simulink model "LQR_simulation"  (R2020b)
settings: Solver=ode45  StartTime=0.0  StopTime=10  FixedStep=0.00001  RelTol=1e-3  EnableMultiTasking=on
values from neighbouring files (symbols this model uses):
  K = lqr(A, B, Q, R)    [LQR.m]
  Theta1_0 = 0    [LQR.m]    (also in LQR_discrete.m; simulation.m = 3.14159265359)
  Theta2_0 = 0.048    [LQR.m]    (also in LQR_discrete.m = 0.04; simulation.m = -1.57079632679)
  Thetad1_0 = 0    [LQR.m]    (also in LQR_discrete.m; simulation.m)
  Thetad2_0 = 0    [LQR.m]    (also in LQR_discrete.m; simulation.m)
settings Model: Creator=rbabuska  LastModifiedBy=fballast
settings DataIOCC: LimitDataPoints=on  SaveFormat=Array  ReturnWorkspaceOutputs=off  SignalLoggingName=sigsOut
settings OptimizationCC: BooleanDataType=off  ExpressionDepthLimit=2147483647  InitFltsAndDblsToZero=on  LifeSpan=inf
settings DebuggingCC: SaveWithParameterizedLinksMsg=none  SignalResolutionControl=TryResolveAllWithWarning  MultiTaskDSMMsg=warning  MultiTaskCondExecSysMsg=none  AllowSymbolicDim=off  StateNameClashWarn=warning  SFUnexpectedBacktrackingDiag=warning  SFNoUnconditionalDefaultTransitionDiag=warning  SFExecutionAtInitializationDiag=none  ArithmeticOperatorsInVariantConditions=warning
settings HardwareCC: ProdBitPerPointer=32  ProdBitPerSizeT=32  ProdBitPerPtrDiffT=32  ProdLargestAtomicFloat=None  ProdIntDivRoundTo=Undefined  ProdEndianess=Unspecified  ProdWordSize=32  ProdHWDeviceType=32-bit Generic  TargetUnknown=on
settings ModelReferenceCC: PropagateSignalLabelsOutOfModel=off
settings SFSimCC: SimUseLocalCustomCode=off  CustomCodeUndefinedFunction=UseInterfaceOnly
settings RTWCC: RTWUseLocalCustomCode=off
settings CodeAppCC: StateflowObjectComments=on
settings GRTTargetCC: TargetFcnLib=ansi_tfl_tmw.mat  TargetLangStandard=C89/C90 (ANSI)  CombineOutputUpdateFcns=off  GRTInterface=on
settings ConfigComp: CovMetricSettings=dw  CovSaveCumulativeToWorkspaceVar=on  CovSaveSingleToWorkspaceVar=on  CovExternalEMLEnable=off

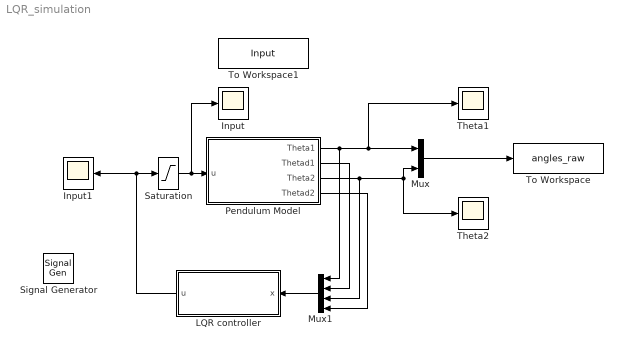
== system LQR_simulation ==
  Input : Scope
  Input1 : Scope
  LQR controller : Subsystem
  Mux : Mux  Inputs=2
  Mux1 : Mux
  Pendulum Model : Subsystem
  Saturation : Saturate  UpperLimit=1  LowerLimit=-1
  Signal Generator : SignalGenerator  Amplitude=0.7  Frequency=3  Units=rad/sec
  Theta1 : Scope
  Theta2 : Scope
  To Workspace : ToWorkspace  VariableName=angles_raw  SaveFormat=Timeseries  SampleTime=-1
  To Workspace1 : ToWorkspace  VariableName=Input  SaveFormat=Timeseries  SampleTime=-1
  wires:
  Pendulum Model/3(Theta2) -> Mux1/3, Mux/2, Theta2/1
  Mux/1 -> To Workspace/1
  Pendulum Model/1(Theta1) -> Mux1/1, Mux/1, Theta1/1
  Pendulum Model/2(Thetad1) -> Mux1/2
  Pendulum Model/4(Thetad2) -> Mux1/4
  Mux1/1 -> LQR controller/1(x)
  LQR controller/1(u) -> Saturation/1, Input1/1
  Saturation/1 -> Input/1, Pendulum Model/1(u)

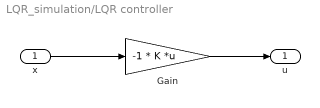
== system LQR_simulation/LQR controller ==
  x : Inport
  Gain : Gain  Gain=-1 * K  Multiplication=Matrix(K*u) (u vector)
  u : Outport
  wires:
  x/1 -> Gain/1
  Gain/1 -> u/1

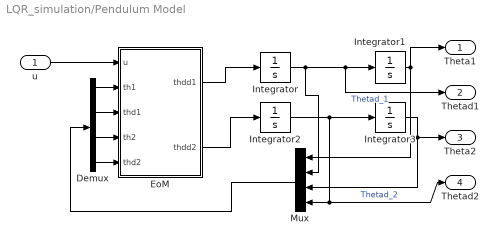
== system LQR_simulation/Pendulum Model ==
  u : Inport
  Demux : Demux
  EoM : MATLAB Function  TreatAsAtomicUnit=on
  Integrator : Integrator  InitialCondition=Thetad1_0  ContinuousStateAttributes='Theta1'
  Integrator1 : Integrator  InitialCondition=Theta1_0  ContinuousStateAttributes='Theta1'
  Integrator2 : Integrator  InitialCondition=Thetad2_0  ContinuousStateAttributes='Theta1'
  Integrator3 : Integrator  InitialCondition=Theta2_0  ContinuousStateAttributes='Theta1'
  Mux : Mux
  Theta1 : Outport
  Thetad1 : Outport  Port=2
  Theta2 : Outport  Port=3
  Thetad2 : Outport  Port=4
  wires:
  Integrator1/1 -> Mux/1, Theta1/1
  Integrator/1 -> Mux/2, Integrator1/1, Thetad1/1  "Thetad_1"
  EoM/2(thdd2) -> Integrator2/1
  Integrator2/1 -> Thetad2/1, Mux/4, Integrator3/1  "Thetad_2"
  Integrator3/1 -> Theta2/1, Mux/3
  u/1 -> EoM/1(u)
  EoM/1(thdd1) -> Integrator/1
  Demux/1 -> EoM/2(th1)
  Demux/2 -> EoM/3(thd1)
  Demux/3 -> EoM/4(th2)
  Demux/4 -> EoM/5(thd2)
  Mux/1 -> Demux/1

== matlab function LQR_simulation/Pendulum Model/EoM ==
  data: u input; thdd1 output; th1 input; thd1 input; th2 input; thd2 input; model_par parameter; thdd2 output
function [thdd1, thdd2] = fcn(u, th1, thd1, th2, thd2, model_par)
thdd1 = -model_par.a11*thd1 - model_par.a12 * u;
F = -model_par.c2*model_par.l1*model_par.m2*sin(thd2)*thd1^2 - model_par.b2*thd2 + model_par.c2*model_par.g*model_par.m2*sin(th1 + th2);
M21 = model_par.m2*model_par.c2^2 + model_par.l1*model_par.m2*cos(thd2)*model_par.c2 + model_par.J2;
M22 = model_par.m2*model_par.c2^2 + model_par.J2;
thdd2 = F/M22 - M21/M22 * thdd1;
